simulink model "systemSim"  (R2021a)
settings: Solver=ode45  StartTime=0.0  StopTime=30  RelTol=1e-5
libraries: simulink x1
settings Model: Creator=alfy  LastModifiedBy=alfy

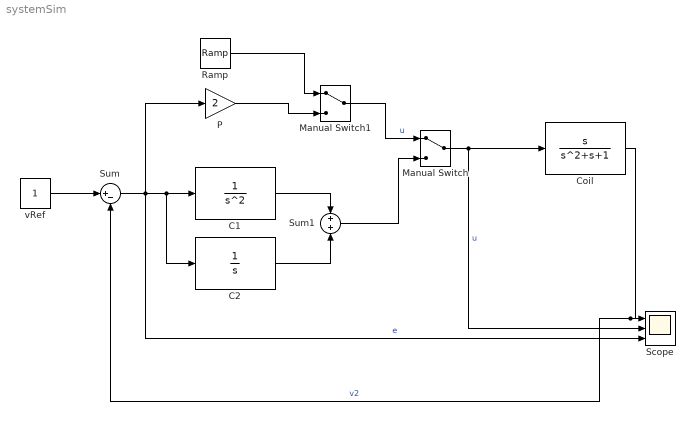
== system systemSim ==
  C1 : TransferFcn  Denominator=[1 0 0]
  C2 : TransferFcn  Denominator=[1 0]
  Coil : TransferFcn  Numerator=[1 0]  Denominator=[1 1 1]
  Manual Switch : ManualSwitch
  Manual Switch1 : ManualSwitch
  P : Gain  Gain=2
  Ramp : simulink/Sources/Ramp  slope=1  start=0  InitialOutput=0
  Scope : Scope  NumInputPorts=3
  Sum : Sum  Inputs=|+-
  Sum1 : Sum  Inputs=+|+
  vRef : Constant
  wires:
  Sum/1 -> P/1, Scope/3, C2/1, C1/1  "e"
  vRef/1 -> Sum/1
  Coil/1 -> Sum/2, Scope/1  "v2"
  Manual Switch/1 -> Scope/2, Coil/1  "u"
  P/1 -> Manual Switch1/2
  C1/1 -> Sum1/1
  C2/1 -> Sum1/2
  Sum1/1 -> Manual Switch/2
  Manual Switch1/1 -> Manual Switch/1  "u"
  Ramp/1 -> Manual Switch1/1
